simulink model "PI_Controller"  (R2020b)
settings: Solver=VariableStepAuto  StartTime=0.0  StopTime=10.0  RelTol=1e-3
values from neighbouring files (symbols this model uses):
  Ki = 45.0    [parameter_data.sldd]
  Kp = 1000.0    [parameter_data.sldd]
settings Model: DataDictionary=parameter_data.sldd  Creator=Vrunda M Balgi  LastModifiedBy=Vrunda M Balgi
settings DataIOCC: SaveOutput=off  SaveTime=off

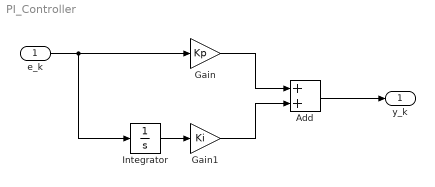
== system PI_Controller ==
  e_k : Inport  OutDataTypeStr=double  PortDimensions=1  SampleTime=0
  Add : Sum
  Gain : Gain  Gain=Kp
  Gain1 : Gain  Gain=Ki
  Integrator : Integrator
  y_k : Outport  OutDataTypeStr=double  PortDimensions=1  SampleTime=0
  wires:
  e_k/1 -> Gain/1, Integrator/1
  Gain/1 -> Add/1
  Gain1/1 -> Add/2
  Integrator/1 -> Gain1/1
  Add/1 -> y_k/1
